simulink model "mdlArchTemplate"  (R2017b)
settings: Solver=FixedStepAuto  StartTime=0.0  StopTime=inf  RelTol=1e-3
PreLoadFcn:
  | myPreloadScript;
values from neighbouring files (symbols this model uses):
  sampleTimeFast = 0.2    [myPreloadScript.m]
undefined symbols (not defined in the file or in its folder): X, Y
libraries: robotlib x4, myAlgorithmLib x2
settings Model: Creator=scastro  LastModifiedBy=scastro
settings OptimizationCC: PassReuseOutputArgsAs=Individual arguments  MaxStackSize=64
settings DebuggingCC: ParameterTunabilityLossMsg=error
settings HardwareCC: ProdBitPerPointer=32  ProdBitPerSizeT=32  ProdBitPerPtrDiffT=32  ProdLargestAtomicFloat=None  ProdIntDivRoundTo=Undefined  ProdEndianess=Unspecified  ProdWordSize=32  ProdHWDeviceType=Generic->Unspecified (assume 32-bit Generic)
settings SFSimCC: MATLABDynamicMemAlloc=off
settings RTWCC: SystemTargetFile=ert.tlc  HardwareBoard=Robot Operating System (ROS)  TemplateMakefile=ert_default_tmf  GenerateReport=on  Toolchain=Catkin  IncludeHyperlinkInReport=on  LaunchReport=on  TargetLang=C++  GenerateTraceInfo=on  GenerateTraceReport=on  GenerateTraceReportSl=on  GenerateTraceReportSf=on  GenerateTraceReportEml=on
settings CodeAppCC: ForceParamTrailComments=on  IgnoreCustomStorageClasses=off  OperatorAnnotations=on  SimulinkDataObjDesc=on  SFDataObjDesc=on  InsertBlockDesc=on

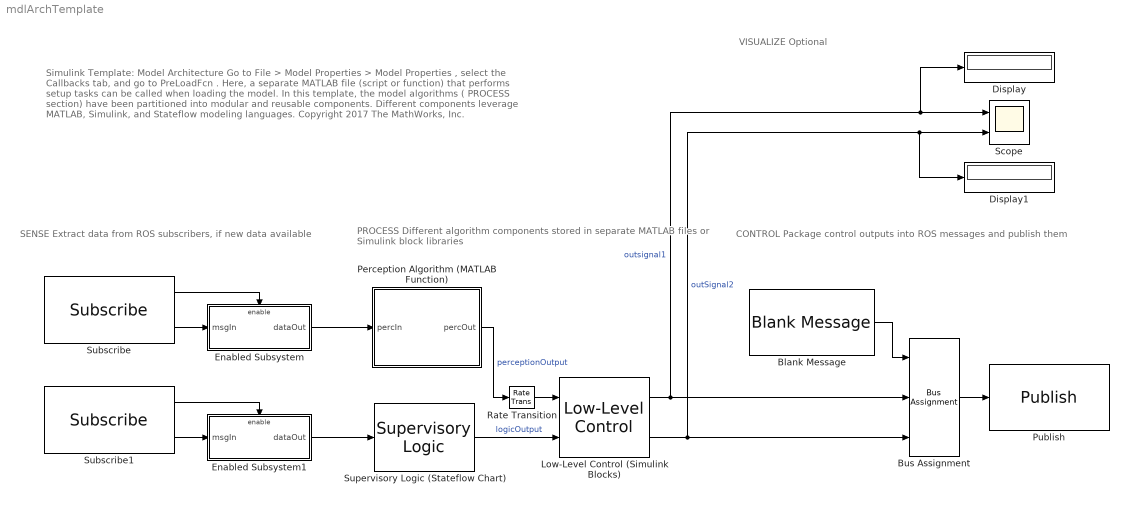
== system mdlArchTemplate ==
  note: PROCESS
      | Different algorithm components stored in
      | separate MATLAB files or Simulink block libraries
  note: SENSE
      | Extract data from ROS subscribers, if new data available
  note: VISUALIZE
      | Optional
  note: CONTROL
      | Package control outputs into ROS messages and publish them
  note: Simulink Template: Model Architecture
      |
      | Go to File > Model Properties > Model Properties , select the Callbacks tab, and go to PreLoadFcn .
      | Here, a separate MATLAB file (script or function) that performs setup tasks can be called when loading the model.
      |
      | In this template, the model algorithms ( PROCESS section) have been partitioned into modular and reusable components. Different components leverage MATLAB, Simulink, and Stateflow modeling languages.
      |
      | Copyright 2017 The MathWorks, Inc.
  Blank Message : robotlib/Blank Message  SourceLibraryInfo=This block requires Robotics System Toolbox  messageType=geometry_msgs/Point  SampleTime=inf
      settings: SourceProductBaseCode=RO
  Bus Assignment : BusAssignment  AssignedSignals=X,Y
  Display : Display
  Display1 : Display
  Enabled Subsystem : Subsystem  TreatAsAtomicUnit=on
  Enabled Subsystem1 : Subsystem  TreatAsAtomicUnit=on
  Low-Level Control (Simulink Blocks) : myAlgorithmLib/Low-Level Control  k1=ctrlParam1  k2=ctrlParam2  Ts=sampleTimeFast
  Perception Algorithm (MATLAB Function) : MATLAB Function  TreatAsAtomicUnit=on
  Publish : robotlib/Publish  SourceLibraryInfo=This block requires Robotics System Toolbox  topicSource=Specify your own  topic=/my_pub_topic  messageType=geometry_msgs/Point  messageQueueLength=1
      settings: SourceProductBaseCode=RO
  Rate Transition : RateTransition
  Scope : Scope  NumInputPorts=2
  Subscribe : robotlib/Subscribe  SourceLibraryInfo=This block requires Robotics System Toolbox  topicSource=Select from ROS network  topic=/my_sub_topic_1  messageType=geometry_msgs/Point  sampleTime=-1  messageQueueLength=1
      settings: SourceProductBaseCode=RO
  Subscribe1 : robotlib/Subscribe  SourceLibraryInfo=This block requires Robotics System Toolbox  topicSource=Select from ROS network  topic=/my_sub_topic_2  messageType=geometry_msgs/Point  sampleTime=-1  messageQueueLength=1
      settings: SourceProductBaseCode=RO
  Supervisory Logic (Stateflow Chart) : myAlgorithmLib/Supervisory Logic
  wires:
  Enabled Subsystem/1(dataOut) -> Perception Algorithm (MATLAB Function)/1(percIn)
  Subscribe/2 -> Enabled Subsystem/1(msgIn)
  Subscribe/1 -> Enabled Subsystem/Enable
  Bus Assignment/1 -> Publish/1
  Blank Message/1 -> Bus Assignment/1
  Low-Level Control (Simulink Blocks)/1 -> Display/1, Scope/1, Bus Assignment/2  "outsignal1"
  Low-Level Control (Simulink Blocks)/2 -> Display1/1, Scope/2, Bus Assignment/3  "outSignal2"
  Subscribe1/1 -> Enabled Subsystem1/Enable
  Subscribe1/2 -> Enabled Subsystem1/1(msgIn)
  Perception Algorithm (MATLAB Function)/1(percOut) -> Rate Transition/1  "perceptionOutput"
  Enabled Subsystem1/1(dataOut) -> Supervisory Logic (Stateflow Chart)/1
  Supervisory Logic (Stateflow Chart)/1 -> Low-Level Control (Simulink Blocks)/2  "logicOutput"
  Rate Transition/1 -> Low-Level Control (Simulink Blocks)/1

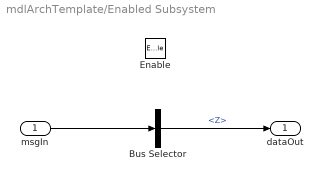
== system mdlArchTemplate/Enabled Subsystem ==
  msgIn : Inport
  Enable : EnablePort
  Bus Selector : BusSelector  OutputSignals=Z
  dataOut : Outport
  wires:
  msgIn/1 -> Bus Selector/1
  Bus Selector/1 -> dataOut/1  "<Z>"

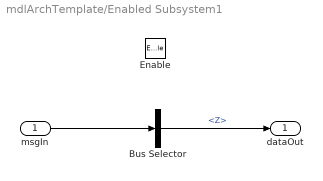
== system mdlArchTemplate/Enabled Subsystem1 ==
  msgIn : Inport
  Enable : EnablePort
  Bus Selector : BusSelector  OutputSignals=Z
  dataOut : Outport
  wires:
  msgIn/1 -> Bus Selector/1
  Bus Selector/1 -> dataOut/1  "<Z>"

== matlab function mdlArchTemplate/Perception Algorithm (MATLAB Function) ==
  settings: updateMethod=DISCRETE  sampleTime=sampleTimeSlow
  data: percIn input; percOut output; perceptionParam parameter
function percOut = perceptionWrapper(percIn, perceptionParam)
% Wrapper function that calls a separate MATLAB file, myPerfectionFcn.m

% The input perceptionParam has been defined as a parameter, which
% references the source workspace. To see data definitions for this
% function, click "Edit Data" in the "Editor" tab of the MATLAB toolstrip.

percOut = myPerceptionFcn(percIn,perceptionParam);
